simulink model "CompoundedDCMachine"  (R2013a)
settings: Solver=ode45  StartTime=0.0  StopTime=0.2  RelTol=1e-3
libraries: powerlib x15, simulink x1
settings Model: Creator=Sony  LastModifiedBy=Sony

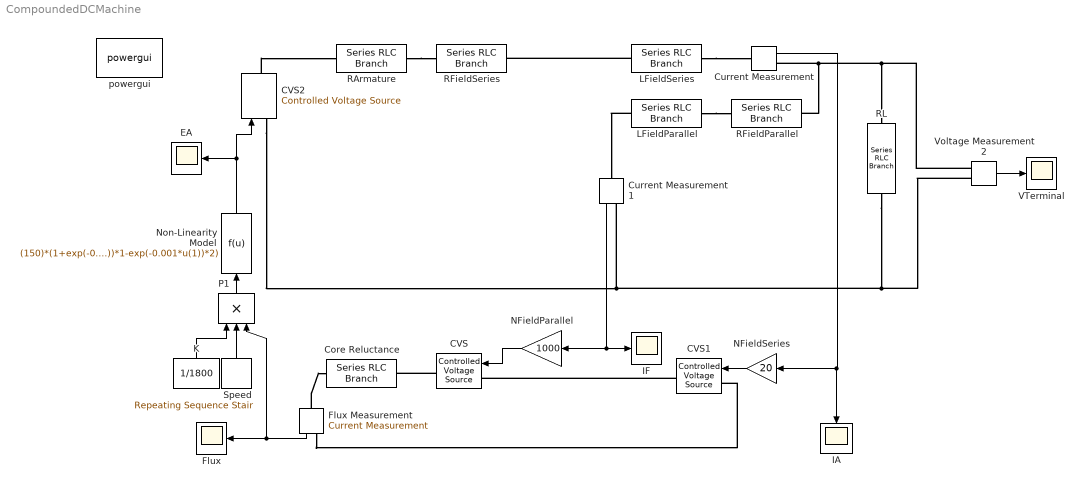
== system CompoundedDCMachine ==
  CVS : powerlib/Electrical Sources/Controlled Voltage Source  Initialize=on  Source_Type=DC  Amplitude=50  Phase=0  Frequency=0  Measurements=None
  CVS1 : powerlib/Electrical Sources/Controlled Voltage Source  Initialize=on  Source_Type=DC  Amplitude=50  Phase=0  Frequency=0  Measurements=None
  CVS2 : powerlib/Electrical Sources/Controlled Voltage Source  Initialize=on  Source_Type=DC  Amplitude=50  Phase=0  Frequency=0  Measurements=None
  Core Reluctance : powerlib/Elements/Series RLC Branch  LConnTagsString=__new0  RConnTagsString=__new0  BranchType=R  Resistance=1  Inductance=1e-3  SetiL0=off  InitialCurrent=0  Capacitance=1e-6  Setx0=off  InitialVoltage=0  Measurements=None
  Current Measurement : powerlib/Measurements/Current Measurement  PhasorSimulation=off  OutputType=Complex  PSBequivalent=0
  Current Measurement1 : powerlib/Measurements/Current Measurement  PhasorSimulation=off  OutputType=Complex  PSBequivalent=0
  EA : Scope
      settings: YMin=0  YMax=120
  Flux : Scope
      settings: YMin=0  YMax=5000  SaveName=ScopeData3
  Flux Measurement : powerlib/Measurements/Current Measurement  PhasorSimulation=off  OutputType=Complex  PSBequivalent=0
  IA : Scope
      settings: YMin=0  YMax=10  SaveName=ScopeData2
  IF : Scope
      settings: YMin=0  YMax=20  SaveName=ScopeData4
  K : Constant  Value=1/1800
  LFieldParallel : powerlib/Elements/Series RLC Branch  LConnTagsString=__new0  RConnTagsString=__new0  BranchType=L  Resistance=30  Inductance=1e-3  SetiL0=on  InitialCurrent=1000  Capacitance=1e-6  Setx0=off  InitialVoltage=0  Measurements=None
  LFieldSeries : powerlib/Elements/Series RLC Branch  LConnTagsString=__new0  RConnTagsString=__new0  BranchType=L  Resistance=0.02  Inductance=1e-3  SetiL0=on  InitialCurrent=1000  Capacitance=1e-6  Setx0=off  InitialVoltage=0  Measurements=None
  NFieldParallel : Gain  Gain=1000
  NFieldSeries : Gain  Gain=20
  Non-Linearity Model : Fcn  Expr=(150)*(1+exp(-0.001*u(1))*1-exp(-0.001*u(1))*2)
  P1 : Product  Inputs=3
  RArmature : powerlib/Elements/Series RLC Branch  LConnTagsString=__new0  RConnTagsString=__new0  BranchType=R  Resistance=0.19  Inductance=1e-3  SetiL0=off  InitialCurrent=0  Capacitance=1e-6  Setx0=off  InitialVoltage=0  Measurements=None
  RFieldParallel : powerlib/Elements/Series RLC Branch  LConnTagsString=__new0  RConnTagsString=__new0  BranchType=R  Resistance=30  Inductance=1e-3  SetiL0=off  InitialCurrent=0  Capacitance=1e-6  Setx0=off  InitialVoltage=0  Measurements=None
  RFieldSeries : powerlib/Elements/Series RLC Branch  LConnTagsString=__new0  RConnTagsString=__new0  BranchType=R  Resistance=0.02  Inductance=1e-3  SetiL0=off  InitialCurrent=0  Capacitance=1e-6  Setx0=off  InitialVoltage=0  Measurements=None
  RL : powerlib/Elements/Series RLC Branch  LConnTagsString=__new0  RConnTagsString=__new0  BranchType=R  Resistance=2.5  Inductance=1e-3  SetiL0=on  InitialCurrent=50  Capacitance=1e-6  Setx0=off  InitialVoltage=0  Measurements=None
  Speed : simulink/Sources/Repeating Sequence Stair  OutValues=[200:10:2500].'  tsamp=1e-3  OutMin=[]  OutMax=[]  OutDataTypeStr=double  OutputDataTypeScalingMode=double  OutDataType=fixdt(0,8)  ConRadixGroup=Best Precision: Vector-wise  OutScaling=2^-12
  VTerminal : Scope
      settings: YMin=0  YMax=200
  Voltage Measurement2 : powerlib/Measurements/Voltage Measurement  PhasorSimulation=off  OutputType=Complex  PSBequivalent=0
  powergui : powerlib/powergui  Priority=1  SimulationMode=Continuous  SolverType=Backward Euler  SampleTime=1e-7  frequency=60  SPID=off  DisableSnubberDevices=off  DisableRonSwitches=off  DisableVfSwitches=off  SwTol=0  Interpol=off  DisplayEquations=off  frequencyindice=0  Pbase=100e6  ErrMax=1e-4  Iterations=50  UnitsV=kV  UnitsW=MW  FunctionMessages=off  echomessages=off  HookPort=off  EnableUseOfTLC=off  x0status=steady  RestoreLinks=warning  ResistiveCurrentMeasurement=off  Frange=[0:2:500]  Ylog=off  Xlog=on  ShowGrid=off  save=off  variable=ZData  ZoomFFT=off  StartTime=0.0  cycles=1  DisplayStyle=1  fundamental=60  FreqAxis=off  MaxFrequency=1000  frequencyindicesteady=1  RmsSteady=1  display=off  Ts=0  methode=off
  wires:
  Current Measurement/1 -> IA/1, NFieldSeries/1
  Current Measurement1/1 -> IF/1, NFieldParallel/1
  NFieldParallel/1 -> CVS/1
  NFieldSeries/1 -> CVS1/1
  Flux Measurement/1 -> Flux/1, P1/3
  Non-Linearity Model/1 -> CVS2/1, EA/1
  Voltage Measurement2/1 -> VTerminal/1
  P1/1 -> Non-Linearity Model/1
  K/1 -> P1/1
  Speed/1 -> P1/2
  connections:
  Voltage Measurement2/LConn1 -- RL/RConn1 -- Current Measurement/RConn1 -- RFieldParallel/LConn1
  Voltage Measurement2/LConn2 -- RL/LConn1 -- CVS2/LConn1 -- Current Measurement1/RConn1
  LFieldParallel/RConn1 -- Current Measurement1/LConn1
  RArmature/RConn1 -- RFieldSeries/LConn1
  LFieldSeries/RConn1 -- Current Measurement/LConn1
  CVS2/RConn1 -- RArmature/LConn1
  Flux Measurement/RConn1 -- CVS1/LConn1
  CVS1/RConn1 -- CVS/LConn1
  CVS/RConn1 -- Core Reluctance/RConn1
  LFieldSeries/LConn1 -- RFieldSeries/RConn1
  LFieldParallel/LConn1 -- RFieldParallel/RConn1
  Flux Measurement/LConn1 -- Core Reluctance/LConn1
